simulink model "wide_FM"  (R2020b)
settings: Solver=VariableStepAuto  StartTime=0.0  StopTime=10.0  RelTol=1e-3
undefined symbols (not defined in the file or in its folder): DiscIntNeverNeededParam, fdesignblkfcn, gcbh
libraries: dspvision x3, dspfdesign x2, simulink x1
settings Model: Creator=MinsooKang  LastModifiedBy=MinsooKang

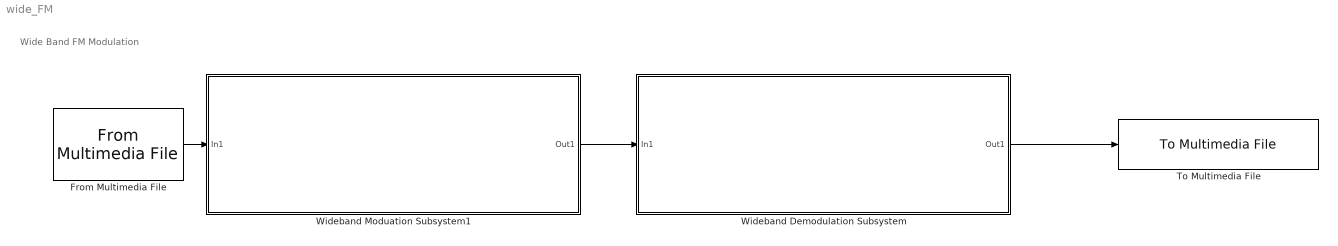
== system wide_FM ==
  note: Wide Band FM Modulation
  From Multimedia File : dspvision/From Multimedia File  inputFilename=C:\Users\MinsooKang\Desktop\matlab\audio.flac  readRange=[1 Inf]  loop=on  numPlays=inf  outputStreams=Audio only  videoDataType=single  audioDataType=double  inheritSampleTime=on  userDefinedSampleTime=1/30  noAudioOutput=off  isIntensityVideo=off  fourcc=RGB  colorVideoFormat=Separate color signals  outputEOF=off  dataOrg=Column-major  audioFrameSize=1  computeAudioFrameSize=off  outSamplingMode=Sample based
  To Multimedia File : dspvision/To Multimedia File  outputFilename=C:\Users\MinsooKang\Desktop\matlab\wide_FM_demodulated.wav  streamSelection=Audio only  videoCompressor=None (uncompressed)  audioCompressor=None (uncompressed)  imagePorts=Separate color signals  fileType=WAV  audioDatatype=32-bit float  fourcc=RGB  videoQuality=75  mj2000CompFactor=10
  Wideband Demodulation Subsystem : Subsystem
  Wideband Moduation Subsystem1 : Subsystem
  wires:
  Wideband Demodulation Subsystem/1(Out1) -> To Multimedia File/1
  From Multimedia File/1 -> Wideband Moduation Subsystem1/1(In1)
  Wideband Moduation Subsystem1/1(Out1) -> Wideband Demodulation Subsystem/1(In1)

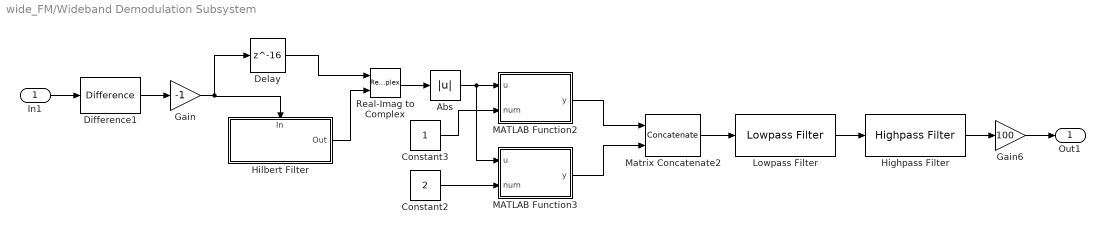
== system wide_FM/Wideband Demodulation Subsystem ==
  In1 : Inport
  Abs : Abs
  Constant2 : Constant  Value=2
  Constant3 : Constant
  Delay : Delay  DelayLength=16  InitialCondition=0
  Difference1 : simulink/Discrete/Difference  ICPrevInput=0.0  OutMin=[]  OutMax=[]  OutDataType=fixdt(1, 16)  OutScaling=2^-10  DoSatur=off
  Gain : Gain  Gain=-1
  Gain6 : Gain  Gain=100
  Highpass Filter : dspfdesign/Highpass Filter  FilterType=FIR  DesignForMinimumOrder=on  FilterOrder=50  StopbandFrequency=20  PassbandFrequency=40  StopbandAttenuation=80  PassbandRipple=0.1  InheritSampleRate=off  SampleRate=44100  SimulateUsing=Interpreted execution  roundingMode=Floor  coeffsDataTypeStr=fixdt(1,16)
  Hilbert Filter : Subsystem  DialogController=fdesignblkfcn  InitFcn=fdesignblkfcn(gcbh, {'InitFcn'});  mask(Hilbert Filter){}
      mask help: Design a Hilbert filter
      settings: CopyFcn=fdesignblkfcn(gcbh, {'CopyFcn'});  PortSchema="{\"entries\":[{\"content\":{\"sides\":[{\"content\":{\"connectorIds\":[]},\"type\":\"ConnectorPlacement.EquallySpacedRectSide\",\"uuid\":\"1b2c5162-6e24-491e-b750-d7b3833c39fb\"},{\"content\":{\"connectorIds\":[\"Out1\"],\"side\":\"RIGHT\"},\"type\":\"ConnectorPlacement.EquallySpacedRectSide\",\"uuid\":\"107a7a6b-a530-42e8-897d-8cd9bd702615\"},{\"content\":{\"connectorIds\":[\"In1\"],\"side\":\"TOP\"},\"type\":\"ConnectorPlacement.EquallySpacedRectSide\",\"uuid\":\"80084fba-0370-4473-bae3-97d3e55bf63e\"},{\"content\":{\"connectorIds\":[],\"side\":\"HIDDEN\"},\"type\":\"ConnectorPlacement.EquallySpacedRectSide\",\"uuid\":\"75b2c584-a684-486d-b930-aceea7921cbc\"}]},\"type\":\"ConnectorPlacement.EquallySpacedConnector\",\"uuid\":\"1e1aa962-7ea9-44b1-8b29-309242de7943\"}],\"packageUris\":[\"http://schema.mathworks.com/mf0/Connector/R2020b\"],\"version\":\"1.0\"}"
      mask Help: helpview(mapfilelocation('dsp'), 'dsphilbertfilter');
      mask Display: disp('Hilbert')
  Lowpass Filter : dspfdesign/Lowpass Filter  FilterType=FIR  DesignForMinimumOrder=on  FilterOrder=50  PassbandFrequency=1500  StopbandFrequency=1600  PassbandRipple=0.1  StopbandAttenuation=80  InheritSampleRate=off  SampleRate=44100  SimulateUsing=Interpreted execution  roundingMode=Floor  coeffsDataTypeStr=fixdt(1,16)
  MATLAB Function2 : MATLAB Function  TreatAsAtomicUnit=on
  MATLAB Function3 : MATLAB Function  TreatAsAtomicUnit=on
  Matrix Concatenate2 : Concatenate  Mode=Multidimensional array  ConcatenateDimension=2
  Real-Imag to Complex : RealImagToComplex
  Out1 : Outport
  wires:
  Matrix Concatenate2/1 -> Lowpass Filter/1
  Difference1/1 -> Gain/1
  Constant3/1 -> MATLAB Function2/2(num)
  MATLAB Function3/1(y) -> Matrix Concatenate2/2
  MATLAB Function2/1(y) -> Matrix Concatenate2/1
  Highpass Filter/1 -> Gain6/1
  Hilbert Filter/1(Out) -> Real-Imag to Complex/2
  Lowpass Filter/1 -> Highpass Filter/1
  Gain/1 -> Delay/1, Hilbert Filter/1(In)
  Abs/1 -> MATLAB Function3/1(u), MATLAB Function2/1(u)
  Delay/1 -> Real-Imag to Complex/1
  Real-Imag to Complex/1 -> Abs/1
  In1/1 -> Difference1/1
  Constant2/1 -> MATLAB Function3/2(num)
  Gain6/1 -> Out1/1

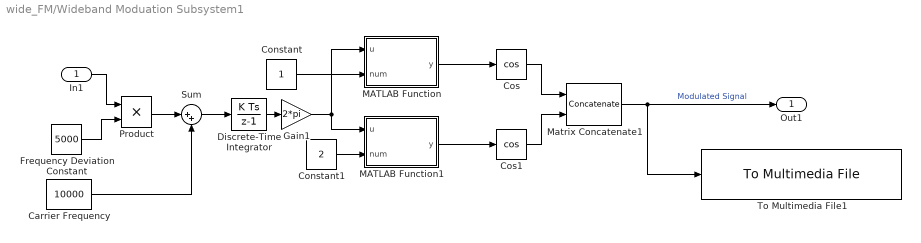
== system wide_FM/Wideband Moduation Subsystem1 ==
  In1 : Inport
  Carrier Frequency : Constant  Value=10000
  Constant : Constant
  Constant1 : Constant  Value=2
  Cos : Trigonometry  Operator=cos
  Cos1 : Trigonometry  Operator=cos
  Discrete-Time Integrator : DiscreteIntegrator  SampleTime=-1  ICPrevOutput=DiscIntNeverNeededParam  ICPrevScaledInput=DiscIntNeverNeededParam
  Frequency Deviation Constant : Constant  Value=5000
  Gain1 : Gain  Gain=2*pi
  MATLAB Function : MATLAB Function  TreatAsAtomicUnit=on
  MATLAB Function1 : MATLAB Function  TreatAsAtomicUnit=on
  Matrix Concatenate1 : Concatenate  Mode=Multidimensional array  ConcatenateDimension=2
  Product : Product
  Sum : Sum  Inputs=|++
  To Multimedia File1 : dspvision/To Multimedia File  outputFilename=C:\Users\MinsooKang\Desktop\matlab\wide_FM_modulated.wav  streamSelection=Audio only  videoCompressor=None (uncompressed)  audioCompressor=None (uncompressed)  imagePorts=Separate color signals  fileType=WAV  audioDatatype=32-bit float  fourcc=RGB  videoQuality=75  mj2000CompFactor=10
  Out1 : Outport
  wires:
  MATLAB Function/1(y) -> Cos/1
  Constant1/1 -> MATLAB Function1/2(num)
  Constant/1 -> MATLAB Function/2(num)
  Frequency Deviation Constant/1 -> Product/2
  Cos/1 -> Matrix Concatenate1/1
  Matrix Concatenate1/1 -> Out1/1, To Multimedia File1/1  "Modulated Signal"
  Cos1/1 -> Matrix Concatenate1/2
  In1/1 -> Product/1
  Carrier Frequency/1 -> Sum/2
  Discrete-Time Integrator/1 -> Gain1/1
  Sum/1 -> Discrete-Time Integrator/1
  Gain1/1 -> MATLAB Function/1(u), MATLAB Function1/1(u)
  MATLAB Function1/1(y) -> Cos1/1
  Product/1 -> Sum/1

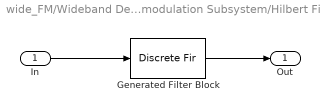
== system wide_FM/Wideband Demodulation Subsystem/Hilbert Filter ==
  In : Inport
  Generated Filter Block : DiscreteFir  Tag=BlockMethodSubSystem  Coefficients=[4.54486433486460064e-05 -0.0319136045611683877 -3.31277815638836425e-05 -0.026047835887445539 -1.5942717018548882e-06 -0.0373284021357406792 3.46942587572346368e-06 -0.0531107459937531778 -1.03378562696822675e-06 -0.0766995375013513336 -5.96683448031529607e-06 -0.116853826766850133 1.66624629077336266e-05 -0.205805810057241412 -1.89302802970533866e-05 -0.634472629392063503 0 0.634472629392063503 1.89302802970533866e-05 0.205805810057241412 -1.66624629077336266e-05 0.116853826766850133 5.96683448031529607e-06 0.0766995375013513336 1.03378562696822675e-06 0.0531107459937531778 -3.46942587572346368e-06 0.0373284021357406792 1.5942717018548882e-06 0.026047835887445539 3.31277815638836425e-05 0.0319136045611683877 -4.54486433486460064e-05]  InputProcessing=Columns as channels (frame based)
  Out : Outport  VectorParamsAs1DForOutWhenUnconnected=off
  wires:
  Generated Filter Block/1 -> Out/1
  In/1 -> Generated Filter Block/1

== matlab function wide_FM/Wideband Moduation Subsystem1/MATLAB Function ==
  data: u input; y output; num input
function y = split(u,num)

y = u(:,num);

== matlab function wide_FM/Wideband Demodulation Subsystem/MATLAB Function2 ==
  data: u input; y output; num input
function y = split(u,num)

y = u(:,num);

== matlab function wide_FM/Wideband Demodulation Subsystem/MATLAB Function3 ==
  data: u input; y output; num input
function y = split(u,num)

y = u(:,num);

== matlab function wide_FM/Wideband Moduation Subsystem1/MATLAB Function1 ==
  data: u input; y output; num input
function y = split(u,num)

y = u(:,num);
